simulink model "lab5"  (R2016b)
settings: Solver=VariableStepAuto  StartTime=0.0  StopTime=30  RelTol=1e-3
libraries: simulink x1
settings Model: Creator=Admin  LastModifiedBy=Admin

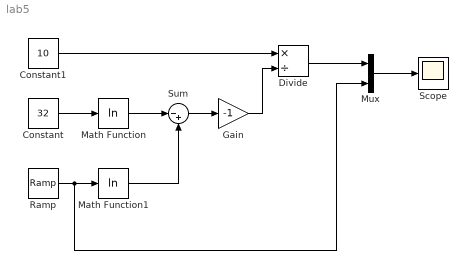
== system lab5 ==
  Constant : Constant  Value=32
  Constant1 : Constant  Value=10
  Divide : Product  Inputs=*/
  Gain : Gain  Gain=-1
  Math Function : Math  Operator=log  SaturateOnIntegerOverflow=on
  Math Function1 : Math  Operator=log  SaturateOnIntegerOverflow=on
  Mux : Mux  Inputs=2
  Ramp : simulink/Sources/Ramp  slope=1  start=0  X0=0
  Scope : Scope
  Sum : Sum  Inputs=|-+
  wires:
  Constant/1 -> Math Function/1
  Math Function/1 -> Sum/1
  Math Function1/1 -> Sum/2
  Sum/1 -> Gain/1
  Gain/1 -> Divide/2
  Constant1/1 -> Divide/1
  Divide/1 -> Mux/1
  Mux/1 -> Scope/1
  Ramp/1 -> Mux/2, Math Function1/1
